simulink model "project_block_diagrams"  (R2020b)
settings: Solver=VariableStepAuto  StartTime=0.0  StopTime=10.0  RelTol=1e-3
undefined symbols (not defined in the file): a, ab, Ci, g, JiCp, Jp, Ki, Kp, l
settings Model: Creator=smutha  LastModifiedBy=smutha

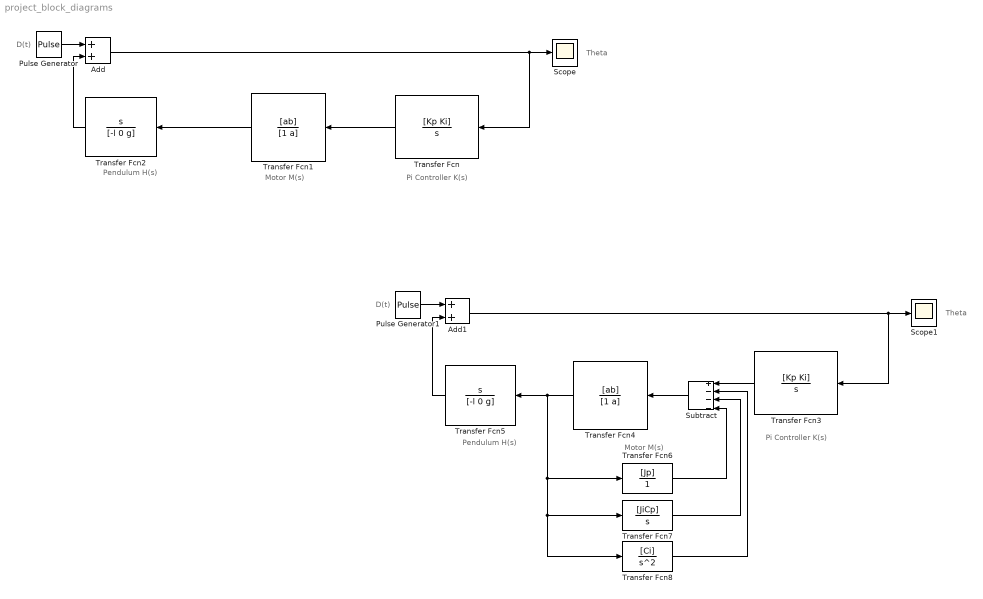
== system project_block_diagrams ==
  note: D(t)
  note: Theta
  note: Pi Controller K(s)
  note: Motor M(s)
  note: Pendulum
      | H(s)
  note: Theta
  note: Pendulum
      | H(s)
  note: Motor M(s)
  note: Pi Controller K(s)
  note: D(t)
  Add : Sum
  Add1 : Sum
  Pulse Generator : DiscretePulseGenerator  PulseType=Time based  Period=10  PulseWidth=5
  Pulse Generator1 : DiscretePulseGenerator  PulseType=Time based  Period=10  PulseWidth=5
  Scope : Scope
  Scope1 : Scope
  Subtract : Sum  Inputs=+---
  Transfer Fcn : TransferFcn  Numerator=[Kp Ki]  Denominator=[1 0]  ContinuousStateAttributes="\"position\""
  Transfer Fcn1 : TransferFcn  Numerator=[ab]  Denominator=[1 a]  ContinuousStateAttributes="\"position\""
  Transfer Fcn2 : TransferFcn  Numerator=[1 0]  Denominator=[-l 0 g]  ContinuousStateAttributes="\"position\""
  Transfer Fcn3 : TransferFcn  Numerator=[Kp Ki]  Denominator=[1 0]  ContinuousStateAttributes="\"position\""
  Transfer Fcn4 : TransferFcn  Numerator=[ab]  Denominator=[1 a]  ContinuousStateAttributes="\"position\""
  Transfer Fcn5 : TransferFcn  Numerator=[1 0]  Denominator=[-l 0 g]  ContinuousStateAttributes="\"position\""
  Transfer Fcn6 : TransferFcn  Numerator=[Jp]  Denominator=[1]
  Transfer Fcn7 : TransferFcn  Numerator=[JiCp]  Denominator=[1 0]
  Transfer Fcn8 : TransferFcn  Numerator=[Ci]  Denominator=[1 0 0]
  wires:
  Pulse Generator/1 -> Add/1
  Add/1 -> Transfer Fcn/1, Scope/1
  Transfer Fcn2/1 -> Add/2
  Transfer Fcn/1 -> Transfer Fcn1/1
  Transfer Fcn1/1 -> Transfer Fcn2/1
  Transfer Fcn3/1 -> Subtract/1
  Pulse Generator1/1 -> Add1/1
  Add1/1 -> Transfer Fcn3/1, Scope1/1
  Transfer Fcn5/1 -> Add1/2
  Transfer Fcn6/1 -> Subtract/4
  Transfer Fcn7/1 -> Subtract/3
  Transfer Fcn8/1 -> Subtract/2
  Subtract/1 -> Transfer Fcn4/1
  Transfer Fcn4/1 -> Transfer Fcn6/1, Transfer Fcn8/1, Transfer Fcn7/1, Transfer Fcn5/1
